simulink model "CH06_5"  (R2019a)
settings: Solver=VariableStepAuto  StartTime=0.0  StopTime=100000000000000000  RelTol=1e-3
libraries: simulink x1
settings Model: Creator=吳俊逸  LastModifiedBy=吳俊逸

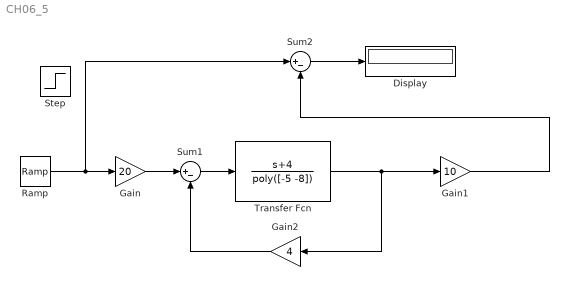
== system CH06_5 ==
  Display : Display
  Gain : Gain  Gain=20
  Gain1 : Gain  Gain=10
  Gain2 : Gain  Gain=4
  Ramp : simulink/Sources/Ramp  slope=5  start=0  InitialOutput=0
  Step : Step  Time=0  After=5  SampleTime=0
  Sum1 : Sum  Inputs=|+-
  Sum2 : Sum  Inputs=|+-
  Transfer Fcn : TransferFcn  Numerator=[1 4]  Denominator=poly([-5 -8])
  wires:
  Sum1/1 -> Transfer Fcn/1
  Gain2/1 -> Sum1/2
  Gain/1 -> Sum1/1
  Ramp/1 -> Gain/1, Sum2/1
  Sum2/1 -> Display/1
  Transfer Fcn/1 -> Gain1/1, Gain2/1
  Gain1/1 -> Sum2/2
